simulink model "envelope analysis_simulink"  (R2020a)
settings: Solver=FixedStepDiscrete  StartTime=0.0  StopTime=inf  RelTol=1e-3
values from neighbouring files (symbols this model uses):
  fs = 48e3    (= 48000)    [bearing_sim.m]    (also in demodulation.m)
undefined symbols (not defined in the file or in its folder): fdesignblkfcn, gcbh
libraries: dspfdesign x2, dspsrcs4 x1, dspsigops x1
settings Model: Creator=holge  LastModifiedBy=holge
settings SolverCC: AutoInsertRateTranBlk=on
settings DataIOCC: LimitDataPoints=on  SaveOutput=off  SignalLogging=off  SaveTime=off
settings OptimizationCC: LifeSpan=inf  SimCompilerOptimization=on
settings DebuggingCC: AlgebraicLoopMsg=error  SingleTaskRateTransMsg=error  AllowSymbolicDim=off  SFUnexpectedBacktrackingDiag=warning  SFNoUnconditionalDefaultTransitionDiag=warning  SFExecutionAtInitializationDiag=none  ArithmeticOperatorsInVariantConditions=warning
settings SFSimCC: SimUseLocalCustomCode=off  CustomCodeUndefinedFunction=UseInterfaceOnly
settings RTWCC: RTWUseLocalCustomCode=off
settings CodeAppCC: StateflowObjectComments=on
settings GRTTargetCC: TargetLangStandard=C89/C90 (ANSI)
settings ConfigComp: CovMetricSettings=dw  CovHtmlReporting=on  CovSaveCumulativeToWorkspaceVar=on  CovSaveSingleToWorkspaceVar=on  CovExternalEMLEnable=off  CovSFcnEnable=off

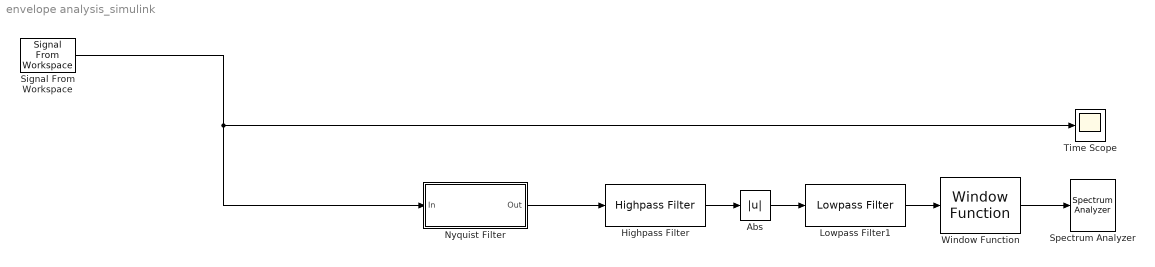
== system envelope analysis_simulink ==
  Abs : Abs
  Highpass Filter : dspfdesign/Highpass Filter  FilterType=FIR  DesignForMinimumOrder=on  FilterOrder=50  StopbandFrequency=100  PassbandFrequency=500  StopbandAttenuation=80  PassbandRipple=0.1  InheritSampleRate=on  SampleRate=fs  SimulateUsing=Interpreted execution  roundingMode=Floor  coeffsDataTypeStr=fixdt(1,16)
  Lowpass Filter1 : dspfdesign/Lowpass Filter  FilterType=FIR  DesignForMinimumOrder=on  FilterOrder=50  PassbandFrequency=1e3  StopbandFrequency=1.2e3  PassbandRipple=0.1  StopbandAttenuation=80  InheritSampleRate=on  SampleRate=44100  SimulateUsing=Interpreted execution  roundingMode=Floor  coeffsDataTypeStr=fixdt(1,16)
  Nyquist Filter : Subsystem  DialogController=fdesignblkfcn  InitFcn=fdesignblkfcn(gcbh, {'InitFcn'});  mask(Nyquist Filter){}
      mask help: Design a Nyquist filter
      settings: CopyFcn=fdesignblkfcn(gcbh, {'CopyFcn'});
      mask Help: helpview(mapfilelocation('dsp'), 'dspnyquistfilter');
      mask Display: disp('Nyquist');
  Signal From Workspace : dspsrcs4/Signal From Workspace  X=xBper  Ts=1/fs  nsamps=1  OutputAfterFinalValue=Cyclic repetition  ignoreOrWarnInputAndFrameLengths=off  OutputFrames=off
  Spectrum Analyzer : SpectrumAnalyzer
  Time Scope : Scope
  Window Function : dspsigops/Window Function  winmode=Apply window to input  wintype=Blackman  sampmode=Continuous  samptime=1  N=64  Rs=50  beta=10  winsamp=Symmetric  UserWindow=hamming  OptParams=off  UserParams={'symmetric'}  dataType=double  isSigned=on  wordLen=16  udDataType=sfix(16)  fracBitsMode=Best precision  numFracBits=15  roundingMode=Floor  overflowMode=off  numSidelobes=4  sidelobeLevel=-30
      settings: SourceProductBaseCode=DS
  wires:
  Signal From Workspace/1 -> Nyquist Filter/1(In), Time Scope/1
  Nyquist Filter/1(Out) -> Highpass Filter/1
  Highpass Filter/1 -> Abs/1
  Abs/1 -> Lowpass Filter1/1
  Lowpass Filter1/1 -> Window Function/1
  Window Function/1 -> Spectrum Analyzer/1

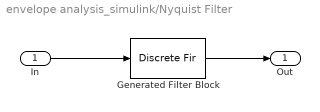
== system envelope analysis_simulink/Nyquist Filter ==
  In : Inport
  Generated Filter Block : DiscreteFir  Tag=BlockMethodSubSystem  Coefficients=[-1.51622726129955863e-05 0 4.17065642797130267e-05 0 -8.63974532359493069e-05 0 0.000156112339412392586 0 -0.000259152163405612895 0 0.000405340967727107018 0 -0.000606122081126900724 0 0.000874664613518894908 0 -0.00122600321576426152 0 0.00167724728876562468 0 -0.00224791534173759749 0 0.00296048017608780203 0 -0.00384125870473808143 0 0.00492186111131599595 0 -0.00624155643186620392 0 0.00785117446710228636 0 -0.00981967458384361454 0 0.0122455627766693432 0 -0.0152776505052993374 0 0.0191551639220552683 0 -0.0242917549435244136 0 0.0314715991488982369 0 -0.0423816072426853388 0 0.0614206608292716463 0 -0.104744991792953324 0 0.317854846111936151 0.5 0.317854846111936151 0 -0.104744991792953324 0 0.0614206608292716463 0 -0.0423816072426853388 0 0.0314715991488982369 0 -0.0242917549435244136 0 0.0191551639220552683 0 -0.0152776505052993374 0 0.0122455627766693432 0 -0.00981967458384361454 0 0.00785117446710228636 0 -0.00624155643186620392 0 0.00492186111131599595 0 -0.00384125870473808143 0 0.00296048017608780203 0 -0.00224791534173759749 0 0.00167724728876562468 0 -0.00122600321576426152 0 0.000874664613518894908 0 -0.000606122081126900724 0 0.000405340967727107018 0 -0.000259152163405612895 0 0.000156112339412392586 0 -8.63974532359493069e-05 0 4.17065642797130267e-05 0 -1.51622726129955863e-05]  InputProcessing=Columns as channels (frame based)
  Out : Outport  VectorParamsAs1DForOutWhenUnconnected=off
  wires:
  In/1 -> Generated Filter Block/1
  Generated Filter Block/1 -> Out/1
